simulink model "horno_baja_temperatura_estrategias"  (R2015a)
settings: Solver=ode45  StartTime=0.0  StopTime=4000  RelTol=1e-3
libraries: simulink x4
settings Model: Creator=m4v  LastModifiedBy=m4v

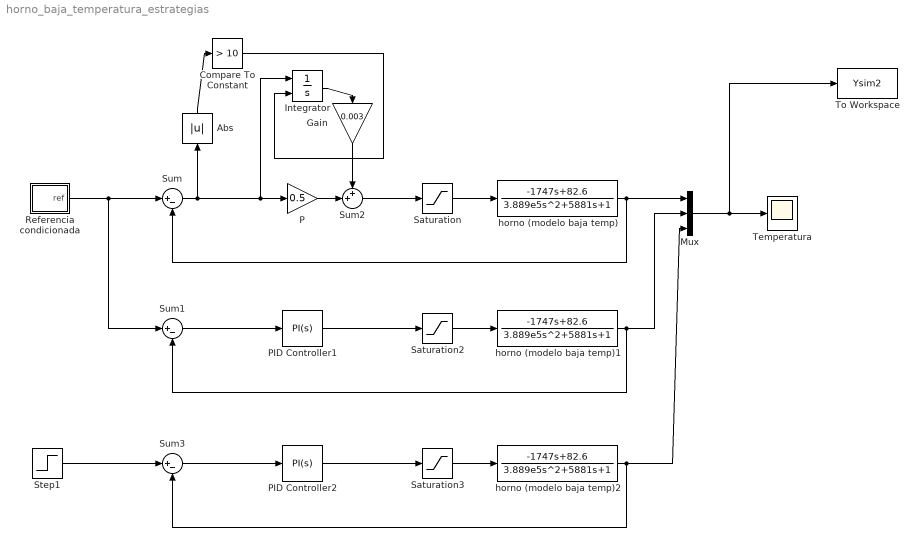
== system horno_baja_temperatura_estrategias ==
  Abs : Abs
  Compare To Constant : simulink/Logic and Bit Operations/Compare To Constant  relop=>  const=10  OutDataTypeStr=boolean
  Gain : Gain  Gain=0.003
  Integrator : Integrator  ExternalReset=level
  Mux : Mux  Inputs=3
  P : Gain  Gain=0.5
  PID Controller1 : simulink/Continuous/PID Controller  Controller=PI  TimeDomain=Continuous-time  SampleTime=-1  IntegratorMethod=Forward Euler  FilterMethod=Forward Euler  Form=Parallel  UseFilter=on  ControllerParametersSource=internal  P=0.5  I=0.0005  D=0  N=100  InitialConditionSource=internal  InitialConditionForIntegrator=0  InitialConditionForFilter=0  ExternalReset=none  LimitOutput=off  UpperSaturationLimit=100  LowerSaturationLimit=0  LinearizeAsGain=on  AntiWindupMode=clamping  Kb=1  TrackingMode=off  Kt=1  PParamMin=[]  PParamMax=[]  IParamMin=[]  IParamMax=[]  DParamMin=[]  DParamMax=[]  NParamMin=[]  NParamMax=[]  KbParamMin=[]  KbParamMax=[]  KtParamMin=[]  KtParamMax=[]  POutMin=[]  POutMax=[]  IOutMin=[]  IOutMax=[]  DOutMin=[]  DOutMax=[]  NOutMin=[]  NOutMax=[]  KbOutMin=[]  KbOutMax=[]  KtOutMin=[]  KtOutMax=[]  IntegratorOutMin=[]  IntegratorOutMax=[]  FilterOutMin=[]  FilterOutMax=[]  SumOutMin=[]  SumOutMax=[]  SumI1OutMin=[]  SumI1OutMax=[]  SumI2OutMin=[]  SumI2OutMax=[]  SumI3OutMin=[]  SumI3OutMax=[]  SumDOutMin=[]  SumDOutMax=[]  SaturationOutMin=[]  SaturationOutMax=[]  IntegratorContinuousStateAttributes=''  IntegratorStateMustResolveToSignalObject=off  IntegratorRTWStateStorageClass=Auto  FilterContinuousStateAttributes=''  FilterStateMustResolveToSignalObject=off  FilterRTWStateStorageClass=Auto  DifferentiatorICPrevScaledInput=0  DifferentiatorOutMin=[]  DifferentiatorOutMax=[]
  PID Controller2 : simulink/Continuous/PID Controller  Controller=PI  TimeDomain=Continuous-time  SampleTime=-1  IntegratorMethod=Forward Euler  FilterMethod=Forward Euler  Form=Parallel  UseFilter=on  ControllerParametersSource=internal  P=0.5  I=0.0005  D=0  N=100  InitialConditionSource=internal  InitialConditionForIntegrator=0  InitialConditionForFilter=0  ExternalReset=none  LimitOutput=off  UpperSaturationLimit=100  LowerSaturationLimit=0  LinearizeAsGain=on  AntiWindupMode=clamping  Kb=1  TrackingMode=off  Kt=1  PParamMin=[]  PParamMax=[]  IParamMin=[]  IParamMax=[]  DParamMin=[]  DParamMax=[]  NParamMin=[]  NParamMax=[]  KbParamMin=[]  KbParamMax=[]  KtParamMin=[]  KtParamMax=[]  POutMin=[]  POutMax=[]  IOutMin=[]  IOutMax=[]  DOutMin=[]  DOutMax=[]  NOutMin=[]  NOutMax=[]  KbOutMin=[]  KbOutMax=[]  KtOutMin=[]  KtOutMax=[]  IntegratorOutMin=[]  IntegratorOutMax=[]  FilterOutMin=[]  FilterOutMax=[]  SumOutMin=[]  SumOutMax=[]  SumI1OutMin=[]  SumI1OutMax=[]  SumI2OutMin=[]  SumI2OutMax=[]  SumI3OutMin=[]  SumI3OutMax=[]  SumDOutMin=[]  SumDOutMax=[]  SaturationOutMin=[]  SaturationOutMax=[]  IntegratorContinuousStateAttributes=''  IntegratorStateMustResolveToSignalObject=off  IntegratorRTWStateStorageClass=Auto  FilterContinuousStateAttributes=''  FilterStateMustResolveToSignalObject=off  FilterRTWStateStorageClass=Auto  DifferentiatorICPrevScaledInput=0  DifferentiatorOutMin=[]  DifferentiatorOutMax=[]
  Referencia condicionada : Subsystem
  Saturation : Saturate  UpperLimit=100  LowerLimit=0  ZeroCross=off
  Saturation2 : Saturate  UpperLimit=100  LowerLimit=0  ZeroCross=off
  Saturation3 : Saturate  UpperLimit=100  LowerLimit=0  ZeroCross=off
  Step1 : Step  After=200  SampleTime=0
  Sum : Sum  Inputs=|+-
  Sum1 : Sum  Inputs=|+-
  Sum2 : Sum  Inputs=++|
  Sum3 : Sum  Inputs=|+-
  Temperatura : Scope
      settings: TimeRange=5000  YMin=-50  YMax=250  SampleInput=on  SampleTime=1
  To Workspace : ToWorkspace  VariableName=Ysim2  SaveFormat=Timeseries  SampleTime=1
  horno (modelo baja temp) : TransferFcn  Numerator=[-1747 82.6]  Denominator=[3.889e5 5881 1]
  horno (modelo baja temp)1 : TransferFcn  Numerator=[-1747 82.6]  Denominator=[3.889e5 5881 1]
  horno (modelo baja temp)2 : TransferFcn  Numerator=[-1747 82.6]  Denominator=[3.889e5 5881 1]
  wires:
  Mux/1 -> To Workspace/1, Temperatura/1
  horno (modelo baja temp)/1 -> Sum/2, Mux/1
  Sum2/1 -> Saturation/1
  Saturation/1 -> horno (modelo baja temp)/1
  P/1 -> Sum2/2
  Integrator/1 -> Gain/1
  Gain/1 -> Sum2/1
  Abs/1 -> Compare To Constant/1
  Compare To Constant/1 -> Integrator/2
  Sum/1 -> Abs/1, P/1, Integrator/1
  horno (modelo baja temp)1/1 -> Mux/2, Sum1/2
  Step1/1 -> Sum3/1
  Saturation2/1 -> horno (modelo baja temp)1/1
  Sum1/1 -> PID Controller1/1
  PID Controller1/1 -> Saturation2/1
  horno (modelo baja temp)2/1 -> Mux/3, Sum3/2
  Saturation3/1 -> horno (modelo baja temp)2/1
  Sum3/1 -> PID Controller2/1
  PID Controller2/1 -> Saturation3/1
  Referencia condicionada/1(ref) -> Sum1/1, Sum/1

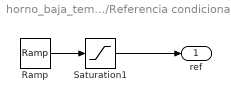
== system horno_baja_temperatura_estrategias/Referencia condicionada ==
  Ramp : simulink/Sources/Ramp  slope=0.3333  start=0  X0=0
  Saturation1 : Saturate  UpperLimit=200  LowerLimit=0
  ref : Outport
  wires:
  Ramp/1 -> Saturation1/1
  Saturation1/1 -> ref/1
